simulink model "EvReferenceApplication"  (R2022b)
settings: Solver=FixedStepAuto  StartTime=0  StopTime=inf  FixedStep=TsEV  RelTol=1e-3  EnableMultiTasking=on
StartFcn:
  | load_system('joystick');
  | set_param('joystick', 'SimulationCommand', 'start');
StopFcn:
  | set_param('joystick', 'SimulationCommand', 'stop');
  | % close_system('joystick')
undefined symbols (not defined in the file or in its folder): DiscIntNeverNeededParam, SRE, TsELEC
libraries: simulink x3, autolibshared x2, autolibutils x1, slrealtimeiplib x1, slrealtimeutilitieslib x1
(part 3 of 3)

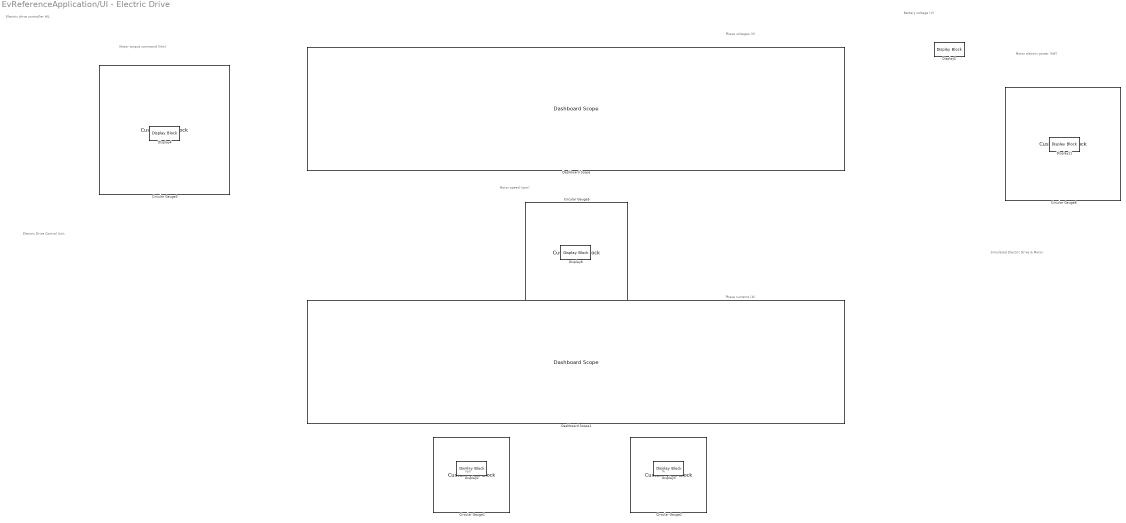
== system EvReferenceApplication/UI - Electric Drive ==
  note: Electric drive controller HIL
  note: kph
  note: %
  note: Motor torque command (Nm)
  note: Phase voltages (V)
  note: Motor speed (rpm)
  note: Battery
      | voltage (V)
  note: Electric Drive
      | Control Unit
  note: Simulated Electric Drive & Motor
  note: Motor electric
      | power (kW)
  note: Phase currents (A)
  Circular Gauge1 : CustomWebBlock  LabelPosition=Hide  ShowInitialText=on  Configuration="{\"components\":[{\"name\":\"CircularScaleComponent\",\"settings\":{\"bounds\":{\"max\":100,\"min\":0,\"tickInterval\":\"auto\"},\"direction\":\"cw\",\"flipLimits\":0,\"innerRadius\":0.75,\"internalTickHeightScaleFactor\":1,\"labelColor\":[228,230,229],\"labelFont\":{\"font\":\"Arial\",\"fontSize\":12},\"labelRadius\":0.528,\"labelTransparency\":1,\"minorTickHeightScaleFactor\":0.2,\"needleImage\":{\"size\":[0,0],\"src\":\"\"},\"needleOffset\":[0,0],\"needleOrientation\":-45,\"needleRotation\":0,\"needleSize\":{\"height\":0,\"width\":0},\"outerRadius\":0.9,\"position\":[0.06486742424242424,0.05627705627705628,0.8917748917748918,0.8787878787878788],\"referencePoint\":\"auto\",\"scaleAngle\":270,\"scaleAngleOffset\":135,\"scaleColors\":[],\"scaleColorsSize\":0.2,\"scaleDirection\":\"CW\",\"scalePosition\":[0,0,1,1],\"showLabels\":1,\"showMinorTicks\":1,\"showSpanLine\":true,\"showTicks\":false,\"tickColor\":[38,38,38],\"tickTransparency\":1,\"valueBarColor\":[0,114,189],\"valueBarPosition\":[0,0,1,1],\"valueBarSize\":0.2,\"valueBarTransparency\":1}},{\"name\":\"BackgroundImageComponent\",\"settings\":{\"image\":{\"size\":[0,0],\"src\":\"default\"},\"position\":[0,0,1,1],\"scaleMode\":\"0\"}},{\"name\":\"ForegroundImageComponent\",\"settings\":{\"image\":{\"size\":[0,0],\"src\":\"default\",\"srcOrientation\":[]},\"isForeground\":1,\"position\":[0,0,1,1],\"scaleMode\":\"0\"}}],\"settings\":{\"BindingType\":\"signal\",\"aspectRatio\":1.032258064516129,\"backgroundColor\":[0,0,0,\"1\"],\"backgroundOffset\":0.14,\"backgroundOpacity\":1,\"direction\":\"cw\",\"fixedAspectRatio\":\"on\",\"flipLimits\":0,\"orientation\":\"horizontal\",\"showBackgroundColor\":false,\"value\":0,\"version\":\"R2022b\"},\"type\":\"CircularGauge\"}"
  Circular Gauge2 : CustomWebBlock  LabelPosition=Hide  ShowInitialText=on  Configuration="{\"components\":[{\"name\":\"CircularScaleComponent\",\"settings\":{\"bounds\":{\"max\":100,\"min\":0,\"tickInterval\":\"auto\"},\"direction\":\"cw\",\"flipLimits\":0,\"innerRadius\":0.75,\"internalTickHeightScaleFactor\":1,\"labelColor\":[228,230,229],\"labelFont\":{\"font\":\"Arial\",\"fontSize\":12},\"labelRadius\":0.528,\"labelTransparency\":1,\"minorTickHeightScaleFactor\":0.2,\"needleImage\":{\"size\":[0,0],\"src\":\"\"},\"needleOffset\":[0,0],\"needleOrientation\":-45,\"needleRotation\":0,\"needleSize\":{\"height\":0,\"width\":0},\"outerRadius\":0.9,\"position\":[0.06486742424242424,0.05627705627705628,0.8917748917748918,0.8787878787878788],\"referencePoint\":\"auto\",\"scaleAngle\":270,\"scaleAngleOffset\":135,\"scaleColors\":[],\"scaleColorsSize\":0.2,\"scaleDirection\":\"CW\",\"scalePosition\":[0,0,1,1],\"showLabels\":1,\"showMinorTicks\":1,\"showSpanLine\":true,\"showTicks\":false,\"tickColor\":[38,38,38],\"tickTransparency\":1,\"valueBarColor\":[0,114,189],\"valueBarPosition\":[0,0,1,1],\"valueBarSize\":0.2,\"valueBarTransparency\":1}},{\"name\":\"BackgroundImageComponent\",\"settings\":{\"image\":{\"size\":[0,0],\"src\":\"default\"},\"position\":[0,0,1,1],\"scaleMode\":\"0\"}},{\"name\":\"ForegroundImageComponent\",\"settings\":{\"image\":{\"size\":[0,0],\"src\":\"default\",\"srcOrientation\":[]},\"isForeground\":1,\"position\":[0,0,1,1],\"scaleMode\":\"0\"}}],\"settings\":{\"BindingType\":\"signal\",\"aspectRatio\":1.032258064516129,\"backgroundColor\":[0,0,0,\"1\"],\"backgroundOffset\":0.14,\"backgroundOpacity\":1,\"direction\":\"cw\",\"fixedAspectRatio\":\"on\",\"flipLimits\":0,\"orientation\":\"horizontal\",\"showBackgroundColor\":false,\"value\":0,\"version\":\"R2022b\"},\"type\":\"CircularGauge\"}"
  Circular Gauge3 : CustomWebBlock  LabelPosition=Hide  ShowInitialText=on  Configuration="{\"components\":[{\"name\":\"CircularScaleComponent\",\"settings\":{\"bounds\":{\"max\":400,\"min\":-300,\"tickInterval\":\"auto\"},\"direction\":\"cw\",\"flipLimits\":0,\"innerRadius\":0.75,\"internalTickHeightScaleFactor\":1,\"labelColor\":[38,38,38],\"labelFont\":{\"font\":\"Arial\",\"fontSize\":12},\"labelRadius\":0.528,\"labelTransparency\":1,\"minorTickHeightScaleFactor\":0.2,\"needleImage\":{\"size\":[0,0],\"src\":\"\"},\"needleOffset\":[0,0],\"needleOrientation\":-45,\"needleRotation\":0,\"needleSize\":{\"height\":0,\"width\":0},\"outerRadius\":0.9,\"position\":[0.06486742424242424,0.05627705627705628,0.8917748917748918,0.8787878787878788],\"referencePoint\":0,\"scaleAngle\":270,\"scaleAngleOffset\":135,\"scaleColors\":[],\"scaleColorsSize\":0.2,\"scaleDirection\":\"CW\",\"scalePosition\":[0,0,1,1],\"showLabels\":1,\"showMinorTicks\":1,\"showSpanLine\":true,\"showTicks\":false,\"tickColor\":[0,114,189],\"tickTransparency\":1,\"valueBarColor\":[0,114,189],\"valueBarPosition\":[0,0,1,1],\"valueBarSize\":0.2,\"valueBarTransparency\":1}},{\"name\":\"BackgroundImageComponent\",\"settings\":{\"image\":{\"size\":[0,0],\"src\":\"default\"},\"position\":[0,0,1,1],\"scaleMode\":\"0\"}},{\"name\":\"ForegroundImageComponent\",\"settings\":{\"image\":{\"size\":[0,0],\"src\":\"default\",\"srcOrientation\":[]},\"isForeground\":1,\"position\":[0,0,1,1],\"scaleMode\":\"0\"}}],\"settings\":{\"BindingType\":\"signal\",\"aspectRatio\":1.032258064516129,\"backgroundColor\":[0,0,0,\"1\"],\"backgroundOffset\":0.14,\"backgroundOpacity\":1,\"direction\":\"cw\",\"fixedAspectRatio\":\"on\",\"flipLimits\":0,\"orientation\":\"horizontal\",\"showBackgroundColor\":false,\"value\":0,\"version\":\"R2022b\"},\"type\":\"CircularGauge\"}"  CustomBackgroundColor="{\"color\":[0.1568627450980392,0.1607843137254902,0.20784313725490197],\"show\":true}"
  Circular Gauge5 : CustomWebBlock  LabelPosition=Hide  ShowInitialText=on  Configuration="{\"components\":[{\"name\":\"CircularScaleComponent\",\"settings\":{\"bounds\":{\"max\":3000,\"min\":0,\"tickInterval\":\"auto\"},\"direction\":\"cw\",\"flipLimits\":0,\"innerRadius\":0.75,\"internalTickHeightScaleFactor\":1,\"labelColor\":[38,38,38],\"labelFont\":{\"font\":\"Arial\",\"fontSize\":12},\"labelRadius\":0.528,\"labelTransparency\":1,\"minorTickHeightScaleFactor\":0.2,\"needleImage\":{\"size\":[0,0],\"src\":\"\"},\"needleOffset\":[0,0],\"needleOrientation\":-45,\"needleRotation\":0,\"needleSize\":{\"height\":0,\"width\":0},\"outerRadius\":0.9,\"position\":[0.06486430921052631,0.05625,0.891633064516129,0.8785978618421053],\"referencePoint\":\"auto\",\"scaleAngle\":270,\"scaleAngleOffset\":135,\"scaleColors\":[],\"scaleColorsSize\":0.2,\"scaleDirection\":\"CW\",\"scalePosition\":[0,0,1,1],\"showLabels\":1,\"showMinorTicks\":1,\"showSpanLine\":true,\"showTicks\":false,\"tickColor\":[0,114,189],\"tickTransparency\":1,\"valueBarColor\":[0,114,189],\"valueBarPosition\":[0,0,1,1],\"valueBarSize\":0.2,\"valueBarTransparency\":1}},{\"name\":\"BackgroundImageComponent\",\"settings\":{\"image\":{\"size\":[0,0],\"src\":\"default\"},\"position\":[0,0,1,1],\"scaleMode\":\"0\"}},{\"name\":\"ForegroundImageComponent\",\"settings\":{\"image\":{\"size\":[0,0],\"src\":\"default\",\"srcOrientation\":[]},\"isForeground\":1,\"position\":[0,0,1,1],\"scaleMode\":\"0\"}}],\"settings\":{\"BindingType\":\"signal\",\"aspectRatio\":1.032258064516129,\"backgroundColor\":[0,0,0,\"1\"],\"backgroundOffset\":0.14,\"backgroundOpacity\":1,\"direction\":\"cw\",\"fixedAspectRatio\":\"on\",\"flipLimits\":0,\"orientation\":\"horizontal\",\"showBackgroundColor\":false,\"value\":0,\"version\":\"R2022b\"},\"type\":\"CircularGauge\"}"  CustomBackgroundColor="{\"color\":[0.1568627450980392,0.1607843137254902,0.20784313725490197],\"show\":true}"
  Circular Gauge8 : CustomWebBlock  LabelPosition=Hide  ShowInitialText=on  Configuration="{\"components\":[{\"name\":\"CircularScaleComponent\",\"settings\":{\"bounds\":{\"max\":200,\"min\":-100,\"tickInterval\":\"auto\"},\"direction\":\"cw\",\"flipLimits\":0,\"innerRadius\":0.75,\"internalTickHeightScaleFactor\":1,\"labelColor\":[38,38,38],\"labelFont\":{\"font\":\"Arial\",\"fontSize\":12},\"labelRadius\":0.528,\"labelTransparency\":1,\"minorTickHeightScaleFactor\":0.2,\"needleImage\":{\"size\":[0,0],\"src\":\"\"},\"needleOffset\":[0,0],\"needleOrientation\":-45,\"needleRotation\":0,\"needleSize\":{\"height\":0,\"width\":0},\"outerRadius\":0.9,\"position\":[0.06487573099415204,0.0561242816091954,0.8917923850574713,0.8786549707602339],\"referencePoint\":0,\"scaleAngle\":270,\"scaleAngleOffset\":135,\"scaleColors\":[],\"scaleColorsSize\":0.2,\"scaleDirection\":\"CW\",\"scalePosition\":[0,0,1,1],\"showLabels\":1,\"showMinorTicks\":1,\"showSpanLine\":true,\"showTicks\":false,\"tickColor\":[0,114,189],\"tickTransparency\":1,\"valueBarColor\":[0,114,189],\"valueBarPosition\":[0,0,1,1],\"valueBarSize\":0.2,\"valueBarTransparency\":1}},{\"name\":\"BackgroundImageComponent\",\"settings\":{\"image\":{\"size\":[0,0],\"src\":\"default\"},\"position\":[0,0,1,1],\"scaleMode\":\"0\"}},{\"name\":\"ForegroundImageComponent\",\"settings\":{\"image\":{\"size\":[0,0],\"src\":\"default\",\"srcOrientation\":[]},\"isForeground\":1,\"position\":[0,0,1,1],\"scaleMode\":\"0\"}}],\"settings\":{\"BindingType\":\"signal\",\"aspectRatio\":1.032258064516129,\"backgroundColor\":[0,0,0,\"1\"],\"backgroundOffset\":0.14,\"backgroundOpacity\":1,\"direction\":\"cw\",\"fixedAspectRatio\":\"on\",\"flipLimits\":0,\"orientation\":\"horizontal\",\"showBackgroundColor\":false,\"value\":0,\"version\":\"R2022b\"},\"type\":\"CircularGauge\"}"  CustomBackgroundColor="{\"color\":[0.1568627450980392,0.1607843137254902,0.20784313725490197],\"show\":true}"
  Dashboard Scope : DashboardScope  TimeSpan=0.050000000000000003  Ymin=-200  Ymax=200  ScaleAtStop=off  UpdateMode=Scroll
  Dashboard Scope1 : DashboardScope  TimeSpan=0.050000000000000003  Ymin=-700  Ymax=700  ScaleAtStop=off  UpdateMode=Scroll
  Display{2..5,8,11} (6 alike) : DisplayBlock  LabelPosition=Hide  Format=Integer  Transparency=1  Opacity=0

== system EvReferenceApplication/Virtual Vehicle ==
  Controllers : Subsystem
      mask Display: image('SystemControllers.png','center')
  Environment : Subsystem
      mask Display: disp(getString(message('autoblks:autoblkVehMask:environ')))
  Longitudinal Driver : Subsystem  Variant=on  VariantControlMode=label  VariantControl=Variant1  LabelModeActiveChoice=0
      mask Display:
      | if strcmp('1',get_param(gcb,'ActiveVariant'))
      |     disp('Open Loop')
      | else
      |     image('LongitudinalDriver.png','center');
      | end
  Passenger Car : Subsystem
      mask Display: image('PassengerVehicle.png','center')
  User Input : Subsystem
      mask Display: image('SpaceMouse.png'); % Use "Edit Image" on toolstrip to change.
  Visualization : Subsystem
      mask Display: disp(getString(message('autoblks:autoblkVehMask:visual')))
  wires:
  Controllers/1(Ctrl) -> Passenger Car/2(Ctrl)
  Passenger Car/1(VehPlnt) -> Longitudinal Driver/2("Vfdbk "), Controllers/2(VehPlnt), Visualization/1(Veh Bus)
  Environment/1(Environment) -> Passenger Car/1(Env)
  Longitudinal Driver/1(" OpCmds") -> Controllers/1(OpCmds)
  User Input/1(speed_cmd) -> Longitudinal Driver/1("Vref ")

== system EvReferenceApplication/Virtual Vehicle/Controllers ==
  OpCmds : Inport
  VehPlnt : Inport  Port=2
  Powertrain Control Input : Subsystem
  Powertrain Control Module (PCM) : Subsystem
  Powertrain Control Output : Subsystem
  Ctrl : Outport  VectorParamsAs1DForOutWhenUnconnected=off
  wires:
  [PtCtrl] -> Ctrl/1
  [OpCmds] -> Powertrain Control Input/1(OpCmds)
  Powertrain Control Output/1(PtCtrl) -> [PtCtrl]
  [VehPlnt] -> Powertrain Control Input/2(VehPlnt)
  VehPlnt/1 -> [VehPlnt]
  OpCmds/1 -> [OpCmds]
  Powertrain Control Input/1(AccelPdl) -> Powertrain Control Module (PCM)/1(AccCmd)
  Powertrain Control Input/2(DecelPdl) -> Powertrain Control Module (PCM)/2(DecCmd)
  Powertrain Control Input/3(VehSpdFdbk) -> Powertrain Control Module (PCM)/3(VehSpdFdbk)
  Powertrain Control Input/4(MotSpd) -> Powertrain Control Module (PCM)/4(MotSpd)
  Powertrain Control Module (PCM)/1(MotTrqCmd) -> Powertrain Control Output/1(MotTrqCmd)
  Powertrain Control Module (PCM)/2(BrakeCmd) -> Powertrain Control Output/2(BrkCmd)
  Powertrain Control Input/5(BMS_Sensors) -> Powertrain Control Module (PCM)/5(BMS_Sensors)
  Powertrain Control Module (PCM)/3(BMS_Info) -> Powertrain Control Output/3(BMS_Info)
  Powertrain Control Module (PCM)/4(BMS_Cmd) -> Powertrain Control Output/4(BMS_Cmd)

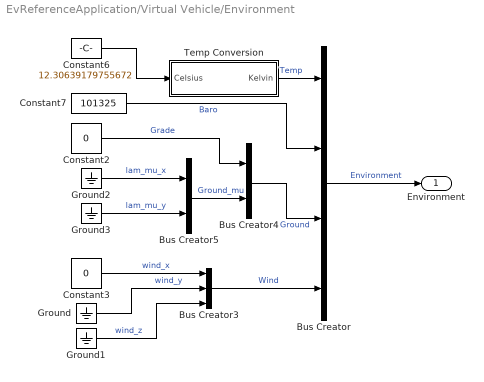
== system EvReferenceApplication/Virtual Vehicle/Environment ==
  Bus Creator : BusCreator  Inputs=4
  Bus Creator3 : BusCreator  Inputs=3
  Bus Creator4 : BusCreator  Inputs=2
  Bus Creator5 : BusCreator  Inputs=2
  Constant2 : Constant  Value=0
  Constant3 : Constant  Value=0
  Constant6 : Constant  Value=12.30639179755672
  Constant7 : Constant  Value=101325
  Ground{,1..3} (4 alike) : Ground
  Temp Conversion : Subsystem
  Environment : Outport  VectorParamsAs1DForOutWhenUnconnected=off
  wires:
  Ground2/1 -> Bus Creator5/1  "lam_mu_x"
  Ground3/1 -> Bus Creator5/2  "lam_mu_y"
  Bus Creator5/1 -> Bus Creator4/2  "Ground_mu"
  Bus Creator4/1 -> Bus Creator/3  "Ground"
  Bus Creator3/1 -> Bus Creator/4  "Wind"
  Constant3/1 -> Bus Creator3/1  "wind_x"
  Ground/1 -> Bus Creator3/2  "wind_y"
  Ground1/1 -> Bus Creator3/3  "wind_z"
  Constant6/1 -> Temp Conversion/1(Celsius)
  Constant2/1 -> Bus Creator4/1  "Grade"
  Bus Creator/1 -> Environment/1  "Environment"
  Constant7/1 -> Bus Creator/2  "Baro"
  Temp Conversion/1(Kelvin) -> Bus Creator/1  "Temp"

== system EvReferenceApplication/Virtual Vehicle/Longitudinal Driver ==
  note: To switch variants, right-click on this subsystem (from one level above) and chose:
      | Variant, Active choice, <your selection>
  "Vref " : Inport
  "Vfdbk " : Inport  Port=2
  Longitudinal Driver : Subsystem  VariantControl=0
      mask Display: image('LongitudinalDriver.png', 'center')
  Open Loop : Subsystem  VariantControl=1
      mask Display: disp('Open Loop')
  " OpCmds" : Outport  VectorParamsAs1DForOutWhenUnconnected=off

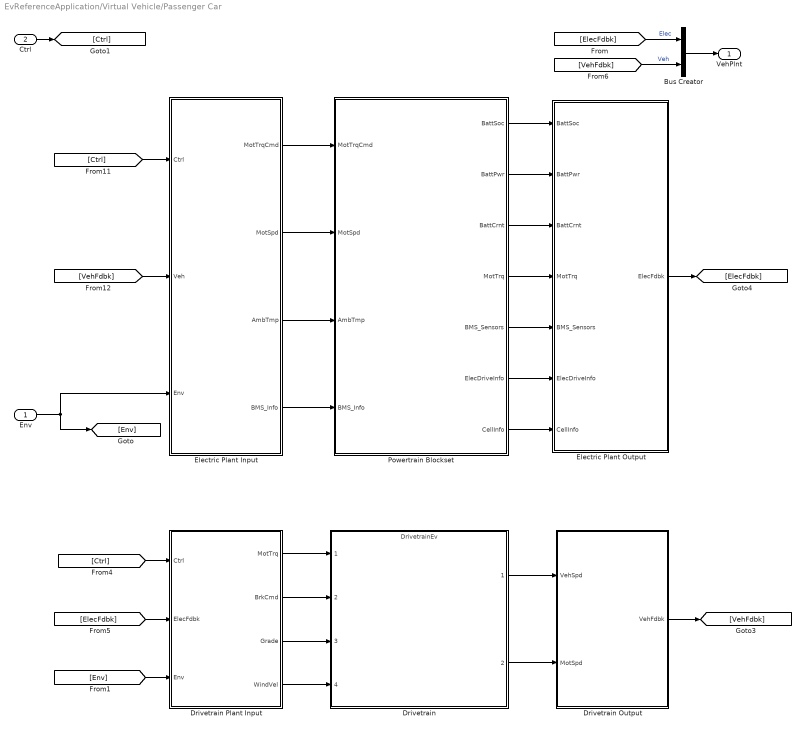
== system EvReferenceApplication/Virtual Vehicle/Passenger Car ==
  Env : Inport
  Ctrl : Inport  Port=2
  Bus Creator : BusCreator  Inputs=2
  Drivetrain : ModelReference  ModelNameDialog=DrivetrainEv.slx  OverrideUsingVariant=Simscape  ModelReferenceVersion=7.0
  Drivetrain Output : Subsystem
  Drivetrain Plant Input : Subsystem
  Electric Plant Input : Subsystem
  Electric Plant Output : Subsystem
  Powertrain Blockset : Subsystem  VariantControl=Powertrain Blockset
  VehPlnt : Outport  VectorParamsAs1DForOutWhenUnconnected=off
  wires:
  Ctrl/1 -> [Ctrl]
  Env/1 -> [Env], Electric Plant Input/3(Env)
  [Ctrl] -> Drivetrain Plant Input/1(Ctrl)
  Bus Creator/1 -> VehPlnt/1
  [VehFdbk] -> Bus Creator/2  "Veh"
  Drivetrain Output/1(VehFdbk) -> [VehFdbk]
  Electric Plant Output/1(ElecFdbk) -> [ElecFdbk]
  [ElecFdbk] -> Bus Creator/1  "Elec"
  [Ctrl] -> Electric Plant Input/1(Ctrl)
  [ElecFdbk] -> Drivetrain Plant Input/2(ElecFdbk)
  [VehFdbk] -> Electric Plant Input/2(Veh)
  Drivetrain Plant Input/2(BrkCmd) -> Drivetrain/2
  Drivetrain Plant Input/1(MotTrq) -> Drivetrain/1
  Drivetrain/2 -> Drivetrain Output/2(MotSpd)
  Drivetrain/1 -> Drivetrain Output/1(VehSpd)
  [Env] -> Drivetrain Plant Input/3(Env)
  Drivetrain Plant Input/3(Grade) -> Drivetrain/3
  Drivetrain Plant Input/4(WindVel) -> Drivetrain/4
  Electric Plant Input/1(MotTrqCmd) -> Powertrain Blockset/1(MotTrqCmd)
  Powertrain Blockset/6(ElecDriveInfo) -> Electric Plant Output/6(ElecDriveInfo)
  Powertrain Blockset/5(BMS_Sensors) -> Electric Plant Output/5(BMS_Sensors)
  Powertrain Blockset/4(MotTrq) -> Electric Plant Output/4(MotTrq)
  Powertrain Blockset/3(BattCrnt) -> Electric Plant Output/3(BattCrnt)
  Powertrain Blockset/2(BattPwr) -> Electric Plant Output/2(BattPwr)
  Powertrain Blockset/1(BattSoc) -> Electric Plant Output/1(BattSoc)
  Electric Plant Input/2(MotSpd) -> Powertrain Blockset/2(MotSpd)
  Electric Plant Input/3(AmbTmp) -> Powertrain Blockset/3(AmbTmp)
  Electric Plant Input/4(BMS_Info) -> Powertrain Blockset/4(BMS_Info)
  Powertrain Blockset/7(CellInfo) -> Electric Plant Output/7(CellInfo)

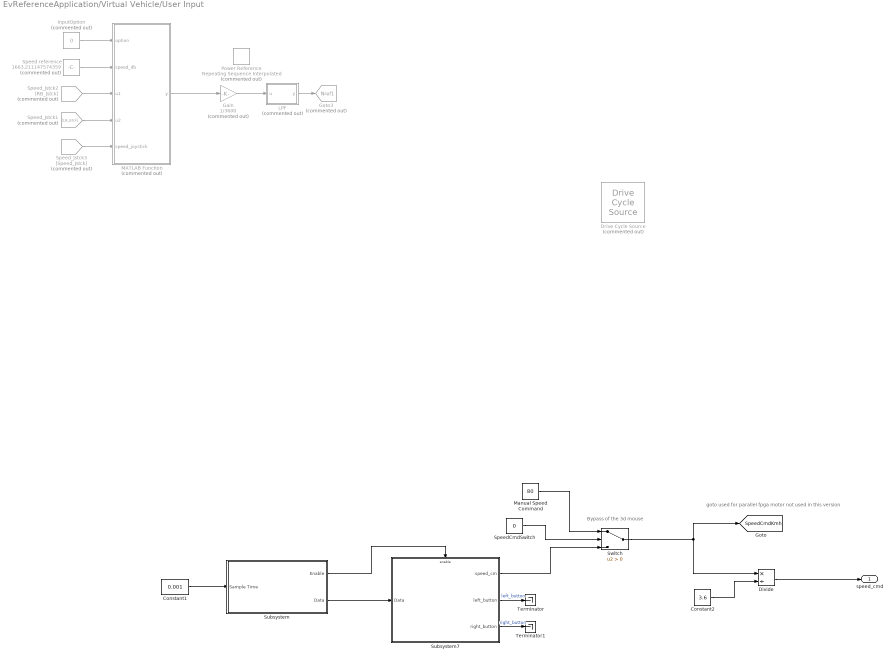
== system EvReferenceApplication/Virtual Vehicle/User Input ==
  note: goto used for parallel fpga motor not used in this version
  note: Bypass of the 3d mouse
  Constant1 : Constant  Value=0.001  SampleTime=0.001
  Constant2 : Constant  Value=3.6  SampleTime=0.001
  Divide : Product  Inputs=*/
  Drive Cycle Source : autolibshared/Drive Cycle Source  Commented=on  cycleVar=FTP75  fileVar=L:\Bauto\matlab\test\toolbox\shared\autoblks\scenario\adac.txt  tfinal="2474  seconds"  cycleRepeat=off  outAccPort=off  outGearPort=off  gearList=No gear data  t_wot1=1  xdot_woto=0  xdot_wot1=26.8*1.1  t_wot2=30  xdot_wot2=0  t_wotend=40  srcUnit=m/s  outUnit=m/s  srcAccUnit=m/s/s  outAccUnit=m/s^2  dt=0  aMode=1  faultOption=off  velBnd=2  velBndUnit=mph  inUnit=m/s  timeBnd=1  failOption=off  stopSim=off  maxFaultCnt=10  maxFaultTime=2  maxTotFaultTime=15  traceOption=off  dtTrace=1  traceWindow=10  lastDCname=FTP75  lastOutUnit=mph  lastDT=0  lastTB=1  lastSB=2  forceCalcBound=off
  Gain : Gain  Commented=on  Gain=1/3600
  Goto3 : Goto  Commented=on  GotoTag=Nref1  TagVisibility=global
  InputOption : Constant  Commented=on  Value=0
  LPF : Subsystem  Commented=on
  MATLAB Function : MATLAB Function  Commented=on  TreatAsAtomicUnit=on
  Manual Speed Command : Constant  Value=80
  Power Reference : simulink/Sources/Repeating Sequence Interpolated  Commented=on  OutValues=[0 0 0.5 0.5 -0.5 -0.5]  TimeValues=[0 5 10 15 25 100]  LookUpMeth=Interpolation-Use End Values  tsamp=TsELEC  OutMin=[]  OutMax=[]  OutDataTypeStr=double  OutputDataTypeScalingMode=double  OutDataType=fixdt(0,8)  OutScaling=2^-10
  Speed reference : Constant  Commented=on  Value=1663.211147574359
  SpeedCmdSwitch : Constant  Value=0
  Speed_Jstck1 : From  Commented=on  GotoTag=LB_Jstck  TagVisibility=global
  Speed_Jstck2 : From  Commented=on  GotoTag=RB_Jstck  TagVisibility=global
  Speed_Jstck3 : From  Commented=on  GotoTag=Speed_Jstck  TagVisibility=global
  Subsystem : Subsystem
  Subsystem7 : Subsystem
  Switch : Switch  Criteria=u2 > Threshold  SaturateOnIntegerOverflow=off  InputSameDT=off
  Terminator : Terminator
  Terminator1 : Terminator
  speed_cmd : Outport
  tag scope: SpeedCmdKmh=global
  wires:
  Gain/1 -> LPF/1(u)
  Speed_Jstck3/1 -> MATLAB Function/5(speed_joystick)
  Subsystem/2(Data) -> Subsystem7/1(Data)
  Constant1/1 -> Subsystem/1(Sample Time)
  Subsystem/1(Enable) -> Subsystem7/Enable
  MATLAB Function/1(y) -> Gain/1
  LPF/1(y) -> Goto3/1
  InputOption/1 -> MATLAB Function/1(option)
  Speed reference/1 -> MATLAB Function/2(speed_db)
  Speed_Jstck2/1 -> MATLAB Function/3(u1)
  Speed_Jstck1/1 -> MATLAB Function/4(u2)
  Subsystem7/2(left_button) -> Terminator/1  "left_button"
  Subsystem7/3(right_button) -> Terminator1/1  "right_button"
  Constant2/1 -> Divide/2
  Divide/1 -> speed_cmd/1
  Manual Speed Command/1 -> Switch/1
  Switch/1 -> [SpeedCmdKmh], Divide/1
  Subsystem7/1(speed_cm) -> Switch/3
  SpeedCmdSwitch/1 -> Switch/2

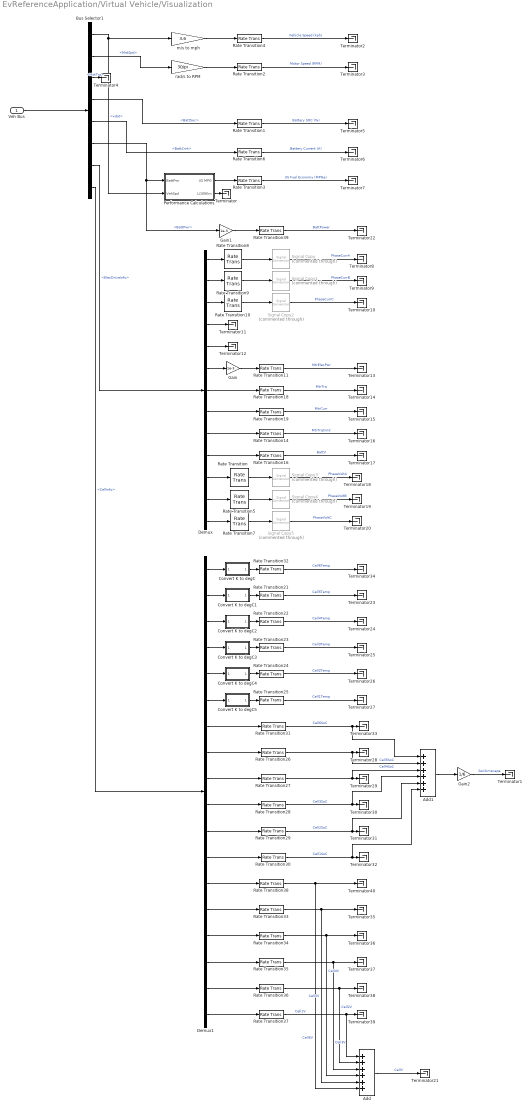
== system EvReferenceApplication/Virtual Vehicle/Visualization ==
  Veh Bus : Inport
  Add : Sum  Inputs=++++++
  Add1 : Sum  Inputs=++++++
  Bus Selector1 : BusSelector  OutputSignals=Veh.xdot,Veh.MotSpd,Elec.MotTrq,Elec.BattSoc,Elec.BattCrnt,Elec.BattPwr,Elec.ElecDriveInfo,Elec.CellInfo
  Convert K to degC : Subsystem
  Convert K to degC1 : Subsystem
  Convert K to degC2 : Subsystem
  Convert K to degC3 : Subsystem
  Convert K to degC4 : Subsystem
  Convert K to degC5 : Subsystem
  Demux : Demux  Outputs=13
  Demux1 : Demux  Outputs=18
  Gain : Gain  Gain=1e-3
  Gain1 : Gain  Gain=1e-3
  Gain2 : Gain  Gain=1/6
  Performance Calculations : Subsystem
  Rate Transition{,5,7..10} (6 alike) : RateTransition  OutPortSampleTime=TsIntrument1kHz
  Rate Transition{1..4,6,11,14,16,18..19} (10 alike) : RateTransition  Deterministic=off  OutPortSampleTime=TsIntrument100Hz
  Rate Transition{21..39} (19 alike) : RateTransition  Deterministic=off  OutPortSampleTime=TsIntrument10Hz
  Signal Copy{,1..5} (6 alike) : SignalConversion  Commented=through  OverrideOpt=on
  Terminator{,1..40} (41 alike) : Terminator
  m/s to mph : Gain  Gain=3.6
  rad/s to RPM : Gain  Gain=30/pi
  wires:
  Bus Selector1/1 -> m/s to mph/1, Performance Calculations/2(VehSpd)  "<xdot>"
  Performance Calculations/1(US MPG) -> Rate Transition3/1
  Performance Calculations/2(L/100Km) -> Terminator/1
  m/s to mph/1 -> Rate Transition4/1
  Bus Selector1/4 -> Rate Transition1/1  "<BattSoc>"
  Rate Transition1/1 -> Terminator5/1  "Battery SOC (%)"
  Rate Transition2/1 -> Terminator3/1  "Motor Speed (RPM)"
  Rate Transition4/1 -> Terminator2/1  "Vehicle Speed (kph)"
  Bus Selector1/2 -> rad/s to RPM/1  "<MotSpd>"
  Bus Selector1/6 -> Gain1/1, Performance Calculations/1(BattPwr)  "<BattPwr>"
  rad/s to RPM/1 -> Rate Transition2/1
  Rate Transition6/1 -> Terminator6/1  "Battery Current (A)"
  Bus Selector1/5 -> Rate Transition6/1  "<BattCrnt>"
  Rate Transition3/1 -> Terminator7/1  "US Fuel Economy (MPGe)"
  Bus Selector1/7 -> Demux/1  "<ElecDriveInfo>"
  Demux/6 -> Gain/1
  Demux/8 -> Rate Transition19/1
  Demux/9 -> Rate Transition14/1
  Demux/1 -> Rate Transition8/1
  Demux/2 -> Rate Transition9/1
  Demux/3 -> Rate Transition10/1
  Rate Transition11/1 -> Terminator13/1  "MtrElecPwr"
  Rate Transition18/1 -> Terminator14/1  "MtrTrq"
  Rate Transition19/1 -> Terminator15/1  "MtrCurr"
  Rate Transition14/1 -> Terminator16/1  "MtrTrqCmd"
  Rate Transition16/1 -> Terminator17/1  "BattV"
  Demux/10 -> Rate Transition16/1
  Demux/11 -> Rate Transition/1
  Demux/12 -> Rate Transition5/1
  Demux/13 -> Rate Transition7/1
  Demux/7 -> Rate Transition18/1
  Gain/1 -> Rate Transition11/1
  Rate Transition32/1 -> Terminator34/1  "Cell6Temp"
  Demux1/1 -> Convert K to degC/1(Kelvin)
  Demux1/2 -> Convert K to degC1/1(Kelvin)
  Rate Transition21/1 -> Terminator23/1  "Cell5Temp"
  Rate Transition22/1 -> Terminator24/1  "Cell4Temp"
  Demux1/3 -> Convert K to degC2/1(Kelvin)
  Demux1/4 -> Convert K to degC3/1(Kelvin)
  Rate Transition23/1 -> Terminator25/1  "Cell3Temp"
  Rate Transition24/1 -> Terminator26/1  "Cell2Temp"
  Demux1/5 -> Convert K to degC4/1(Kelvin)
  Demux1/6 -> Convert K to degC5/1(Kelvin)
  Rate Transition25/1 -> Terminator27/1  "Cell1Temp"
  Rate Transition30/1 -> Add1/6, Terminator32/1  "Cell1SoC"
  Demux1/12 -> Rate Transition30/1
  Demux1/11 -> Rate Transition29/1
  Rate Transition29/1 -> Add1/5, Terminator31/1  "Cell2SoC"
  Rate Transition28/1 -> Add1/4, Terminator30/1  "Cell3SoC"
  Demux1/10 -> Rate Transition28/1
  Demux1/9 -> Rate Transition27/1
  Rate Transition27/1 -> Add1/3, Terminator29/1  "Cell4SoC"
  Rate Transition26/1 -> Add1/2, Terminator28/1  "Cell5SoC"
  Demux1/8 -> Rate Transition26/1
  Demux1/7 -> Rate Transition31/1
  Rate Transition31/1 -> Add1/1, Terminator33/1  "Cell6SoC"
  Rate Transition38/1 -> Add/6, Terminator40/1  "Cell6V"
  Demux1/13 -> Rate Transition38/1
  Demux1/14 -> Rate Transition33/1
  Rate Transition33/1 -> Add/5, Terminator35/1  "Cell5V"
  Rate Transition34/1 -> Add/4, Terminator36/1  "Cell4V"
  Demux1/15 -> Rate Transition34/1
  Demux1/16 -> Rate Transition35/1
  Rate Transition35/1 -> Add/3, Terminator37/1  "Cell3V"
  Rate Transition36/1 -> Add/2, Terminator38/1  "Cell2V"
  Demux1/17 -> Rate Transition36/1
  Demux1/18 -> Rate Transition37/1
  Rate Transition37/1 -> Add/1, Terminator39/1  "Cell1V"
  Bus Selector1/8 -> Demux1/1  "<CellInfo>"
  Convert K to degC/1(Out1) -> Rate Transition32/1
  Convert K to degC1/1(Out1) -> Rate Transition21/1
  Convert K to degC2/1(Out1) -> Rate Transition22/1
  Convert K to degC3/1(Out1) -> Rate Transition23/1
  Convert K to degC4/1(Out1) -> Rate Transition24/1
  Convert K to degC5/1(Out1) -> Rate Transition25/1
  Add/1 -> Terminator21/1  "CellV"
  Gain1/1 -> Rate Transition39/1
  Rate Transition39/1 -> Terminator22/1  "BattPower"
  Bus Selector1/3 -> Terminator4/1  "<MotTrq>"
  Demux/4 -> Terminator11/1
  Demux/5 -> Terminator12/1
  Veh Bus/1 -> Bus Selector1/1
  Signal Copy/1 -> Terminator8/1  "PhaseCurrA"
  Signal Copy1/1 -> Terminator9/1  "PhaseCurrB"
  Signal Copy2/1 -> Terminator10/1  "PhaseCurrC"
  Signal Copy3/1 -> Terminator18/1  "PhaseVoltA"
  Signal Copy4/1 -> Terminator19/1  "PhaseVoltB"
  Signal Copy5/1 -> Terminator20/1  "PhaseVoltC"
  Add1/1 -> Gain2/1
  Gain2/1 -> Terminator1/1  "SocSimscape"
  Rate Transition/1 -> Signal Copy3/1
  Rate Transition5/1 -> Signal Copy4/1
  Rate Transition7/1 -> Signal Copy5/1
  Rate Transition8/1 -> Signal Copy/1
  Rate Transition9/1 -> Signal Copy1/1
  Rate Transition10/1 -> Signal Copy2/1

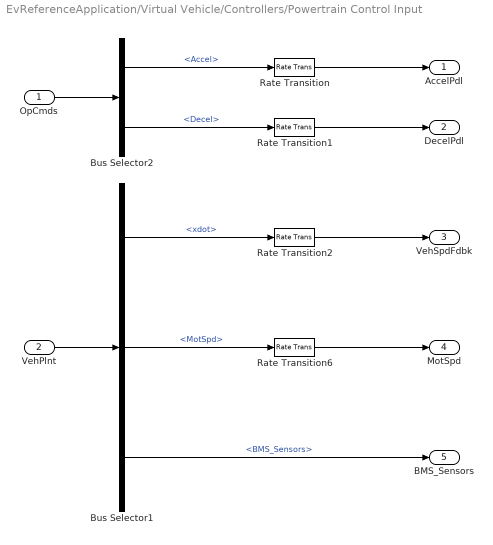
== system EvReferenceApplication/Virtual Vehicle/Controllers/Powertrain Control Input ==
  OpCmds : Inport
  VehPlnt : Inport  Port=2
  Bus Selector1 : BusSelector  OutputSignals=Veh.xdot,Veh.MotSpd,Elec.BMS_Sensors
  Bus Selector2 : BusSelector  OutputSignals=Accel,Decel
  Rate Transition{,1..2,6} (4 alike) : RateTransition  Deterministic=off
  AccelPdl : Outport  VectorParamsAs1DForOutWhenUnconnected=off
  DecelPdl : Outport  Port=2  VectorParamsAs1DForOutWhenUnconnected=off
  VehSpdFdbk : Outport  Port=3  VectorParamsAs1DForOutWhenUnconnected=off
  MotSpd : Outport  Port=4  VectorParamsAs1DForOutWhenUnconnected=off
  BMS_Sensors : Outport  Port=5  OutDataTypeStr=Bus: Sensors  VectorParamsAs1DForOutWhenUnconnected=off
  wires:
  OpCmds/1 -> Bus Selector2/1
  VehPlnt/1 -> Bus Selector1/1
  Bus Selector2/1 -> Rate Transition/1  "<Accel>"
  Bus Selector2/2 -> Rate Transition1/1  "<Decel>"
  Bus Selector1/1 -> Rate Transition2/1  "<xdot>"
  Bus Selector1/2 -> Rate Transition6/1  "<MotSpd>"
  Rate Transition/1 -> AccelPdl/1
  Rate Transition1/1 -> DecelPdl/1
  Rate Transition2/1 -> VehSpdFdbk/1
  Rate Transition6/1 -> MotSpd/1
  Bus Selector1/3 -> BMS_Sensors/1  "<BMS_Sensors>"

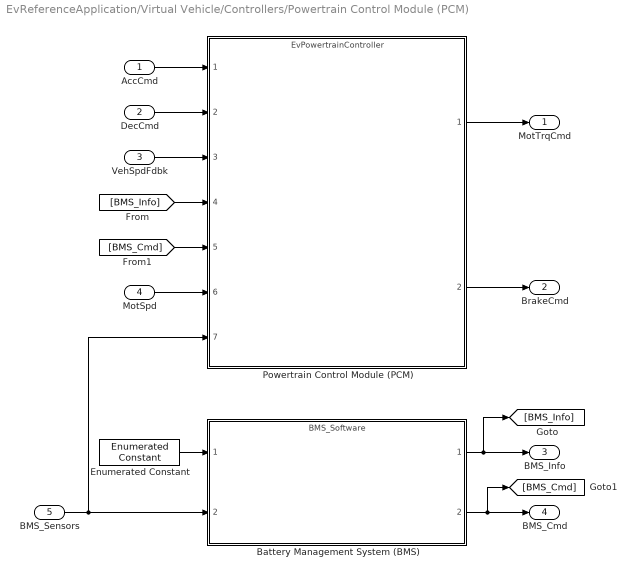
== system EvReferenceApplication/Virtual Vehicle/Controllers/Powertrain Control Module (PCM) ==
  AccCmd : Inport
  DecCmd : Inport  Port=2
  VehSpdFdbk : Inport  Port=3
  MotSpd : Inport  Port=4
  BMS_Sensors : Inport  Port=5  OutDataTypeStr=Bus: Sensors
  Battery Management System (BMS) : ModelReference  ModelNameDialog=BMS_Software.slx  ModelReferenceVersion=4.6
  Enumerated Constant : simulink/Sources/Enumerated Constant  OutDataTypeStr=Enum: SRE  Value=SRE.Driving  SampleTime=inf
  Powertrain Control Module (PCM) : ModelReference  ModelNameDialog=EvPowertrainController.slx  ModelReferenceVersion=5.1
  MotTrqCmd : Outport
  BrakeCmd : Outport  Port=2
  BMS_Info : Outport  Port=3  OutDataTypeStr=Bus: BMS_Info
  BMS_Cmd : Outport  Port=4  OutDataTypeStr=Bus: BMS_Cmd
  wires:
  DecCmd/1 -> Powertrain Control Module (PCM)/2
  Powertrain Control Module (PCM)/1 -> MotTrqCmd/1
  [BMS_Info] -> Powertrain Control Module (PCM)/4
  MotSpd/1 -> Powertrain Control Module (PCM)/6
  VehSpdFdbk/1 -> Powertrain Control Module (PCM)/3
  AccCmd/1 -> Powertrain Control Module (PCM)/1
  Powertrain Control Module (PCM)/2 -> BrakeCmd/1
  Enumerated Constant/1 -> Battery Management System (BMS)/1
  Battery Management System (BMS)/1 -> [BMS_Info], BMS_Info/1
  Battery Management System (BMS)/2 -> [BMS_Cmd], BMS_Cmd/1
  BMS_Sensors/1 -> Powertrain Control Module (PCM)/7, Battery Management System (BMS)/2
  [BMS_Cmd] -> Powertrain Control Module (PCM)/5

== system EvReferenceApplication/Virtual Vehicle/Controllers/Powertrain Control Output ==
  MotTrqCmd : Inport
  BrkCmd : Inport  Port=2
  BMS_Info : Inport  Port=3  OutDataTypeStr=Bus: BMS_Info
  BMS_Cmd : Inport  Port=4  OutDataTypeStr=Bus: BMS_Cmd
  Bus Creator : BusCreator  Inputs=4
  PtCtrl : Outport  VectorParamsAs1DForOutWhenUnconnected=off
  wires:
  BrkCmd/1 -> Bus Creator/2  "BrkCmd"
  Bus Creator/1 -> PtCtrl/1  "PtCtrl"
  MotTrqCmd/1 -> Bus Creator/1  "MotTrqCmd"
  BMS_Info/1 -> Bus Creator/3  "BMS_Info"
  BMS_Cmd/1 -> Bus Creator/4  "BMS_Cmd"

== system EvReferenceApplication/Virtual Vehicle/Environment/Temp Conversion ==
  Celsius : Inport
  Convert degC to K : Subsystem
  Kelvin : Outport
  wires:
  Convert degC to K/1(Out1) -> Kelvin/1
  Celsius/1 -> Convert degC to K/1(Celsius)

== system EvReferenceApplication/Virtual Vehicle/Longitudinal Driver/Longitudinal Driver ==
  Vref : Inport
  Vfdbk : Inport  Port=2
  Bus Selector : BusSelector  OutputSignals=Veh.xdot
  Ground : Ground
  Longitudinal Driver Model : autolibshared/Longitudinal Driver  extAccelOvr=off  extDecelOvr=off  extAccelHld=off  extDecelHld=off  extAccelZero=off  extDecelZero=off  cntrlType=Predictive  shftType=Reverse, Neutral, Drive  velUnits=m/s  gearOut=off  Kp=1  Ki=1  Kff=0  Kg=0  VehVelVec=[0 100]  KffVec=[.1 .1]  KpVec=[10 10]  KiVec=[5 5]  KgVec=[0 0]  m=1645  Kpt=450*9.04/0.324  tau=0.12  L=4  aR=30.3/3875  bR=0.21290*4.44822/0.44704  cR=0.01278*4.44822/0.44704^2  g=9.81  vnom=1  Kaw=0  tauerr=0  tauPt=2  GearInit=0  tShift=.1  pdlVec=[0.1 0.4 0.5 0.9]  upShftTbl=[-1 12.9375 26.4375 39.9375 51.18749999999999 62.4375 72.84375 83.25;-1 16.3125 29.8125 43.3125 54.5624 65.8125 76.78125 87.75;-1 19.6875 33.1875 46.68749999999999 57.9375 69.1875 80.71875 92.25;-1 33 52.5 77.25 100.5 138.75 161.875 185]  dwnShftTbl=[1 9.5625 23.0625 36.5625 47.8125 59.0625 68.90625 78.75;1 12.9375 26.4375 39.9375 51.18749999999999 62.4375 72.84375 83.25;1 16.3125 29.8125 43.3125 54.562499 65.8125 76.78125 87.75;1 19.6875 33.1875 46.68749999999999 57.9375 69.1875 80.71875 92.25]  tClutch=.5  tRev=.5  tPark=120  aMode=1  UpGearVec="[0  1  2  3  4  5  6  7]"  DownGearVec="[1  2  3  4  5  6  7  8]"
  Terminator : Terminator
  Terminator1 : Terminator
  OpCmds : Outport  VectorParamsAs1DForOutWhenUnconnected=off
  wires:
  Bus Selector/1 -> Longitudinal Driver Model/2  "<xdot>"
  Vref/1 -> Longitudinal Driver Model/1  "xdotref"
  Vfdbk/1 -> Bus Selector/1
  Longitudinal Driver Model/2 -> Terminator/1  "Acc"
  Longitudinal Driver Model/3 -> Terminator1/1  "Dec"
  Ground/1 -> Longitudinal Driver Model/3
  Longitudinal Driver Model/1 -> OpCmds/1  "Info"

== system EvReferenceApplication/Virtual Vehicle/Longitudinal Driver/Open Loop ==
  note: This subsystem is provided to disable the driver subsystem and expose the driver interface.
      |
      | The interface can:
      | - be connected with dashboard UI blocks or 3rd party hardware
      | - provide application specific pre-programmed event or time based signals
      | - be driven by recorded operator signals for tuning, troubleshooting and model validation
  Bus Creator2 : BusCreator  Inputs=8
  Constant{1..4} (4 alike) : Constant  Value=0
  Ground{,1..3} (4 alike) : Ground
  OpCmds : Outport  VectorParamsAs1DForOutWhenUnconnected=off
  wires:
  Ground3/1 -> Bus Creator2/8  "ErrMin"
  Ground1/1 -> Bus Creator2/6  "ErrSqrSum"
  Bus Creator2/1 -> OpCmds/1  "Info"
  Ground2/1 -> Bus Creator2/7  "ErrMax"
  Constant1/1 -> Bus Creator2/1  "Accel"
  Constant3/1 -> Bus Creator2/3  "Gear"
  Constant2/1 -> Bus Creator2/2  "Decel"
  Ground/1 -> Bus Creator2/5  "Err"
  Constant4/1 -> Bus Creator2/4  "Clutch"

== system EvReferenceApplication/Virtual Vehicle/Passenger Car/Drivetrain Output ==
  VehSpd : Inport
  MotSpd : Inport  Port=2
  Bus Creator1 : BusCreator  Inputs=2
  VehFdbk : Outport  VectorParamsAs1DForOutWhenUnconnected=off
  wires:
  Bus Creator1/1 -> VehFdbk/1  "VehFdbk"
  VehSpd/1 -> Bus Creator1/1
  MotSpd/1 -> Bus Creator1/2  "MotSpd"

== system EvReferenceApplication/Virtual Vehicle/Passenger Car/Drivetrain Plant Input ==
  Ctrl : Inport
  ElecFdbk : Inport  Port=2
  Env : Inport  Port=3
  Bus Selector : BusSelector  OutputSignals=BrkCmd
  Bus Selector1 : BusSelector  OutputSignals=MotTrq
  Bus Selector3 : BusSelector  OutputSignals=Ground.Grade,Wind.wind_x
  First Order Hold : FirstOrderHold  ErrorTolerance=inf
  Rate Transition6 : RateTransition  Deterministic=off
  Rate Transition7 : RateTransition  Deterministic=off
  MotTrq : Outport  VectorParamsAs1DForOutWhenUnconnected=off
  BrkCmd : Outport  Port=2  VectorParamsAs1DForOutWhenUnconnected=off
  Grade : Outport  Port=3  VectorParamsAs1DForOutWhenUnconnected=off
  WindVel : Outport  Port=4  VectorParamsAs1DForOutWhenUnconnected=off
  wires:
  Ctrl/1 -> Bus Selector/1
  Bus Selector/1 -> First Order Hold/1  "<BrkCmd>"
  First Order Hold/1 -> BrkCmd/1  "BrkCmd"
  ElecFdbk/1 -> Bus Selector1/1
  Bus Selector1/1 -> MotTrq/1  "<MotTrq>"
  Env/1 -> Bus Selector3/1
  Rate Transition6/1 -> Grade/1  "Grade"
  Rate Transition7/1 -> WindVel/1  "WindVel"
  Bus Selector3/1 -> Rate Transition6/1  "<Grade>"
  Bus Selector3/2 -> Rate Transition7/1  "<wind_x>"

== system EvReferenceApplication/Virtual Vehicle/Passenger Car/Electric Plant Input ==
  Ctrl : Inport
  Veh : Inport  Port=2
  Env : Inport  Port=3
  Bus Selector : BusSelector  OutputSignals=MotTrqCmd,BMS_Info
  Bus Selector1 : BusSelector  OutputSignals=MotSpd
  Bus Selector2 : BusSelector  OutputSignals=Temp
  First Order Hold : FirstOrderHold  ErrorTolerance=inf
  MotTrqCmd : Outport  VectorParamsAs1DForOutWhenUnconnected=off
  MotSpd : Outport  Port=2  VectorParamsAs1DForOutWhenUnconnected=off
  AmbTmp : Outport  Port=3  VectorParamsAs1DForOutWhenUnconnected=off
  BMS_Info : Outport  Port=4  OutDataTypeStr=Bus: BMS_Info  VectorParamsAs1DForOutWhenUnconnected=off
  wires:
  First Order Hold/1 -> MotTrqCmd/1  "MotTrqCmd"
  Ctrl/1 -> Bus Selector/1
  Bus Selector/1 -> First Order Hold/1  "<MotTrqCmd>"
  Veh/1 -> Bus Selector1/1
  Bus Selector1/1 -> MotSpd/1  "<MotSpd>"
  Env/1 -> Bus Selector2/1
  Bus Selector2/1 -> AmbTmp/1  "<Temp>"
  Bus Selector/2 -> BMS_Info/1  "<BMS_Info>"

== system EvReferenceApplication/Virtual Vehicle/Passenger Car/Electric Plant Output ==
  BattSoc : Inport
  BattPwr : Inport  Port=2
  BattCrnt : Inport  Port=3
  MotTrq : Inport  Port=4
  BMS_Sensors : Inport  Port=5  OutDataTypeStr=Bus: Sensors
  ElecDriveInfo : Inport  Port=6
  CellInfo : Inport  Port=7
  Bus Creator1 : BusCreator  Inputs=7
  ElecFdbk : Outport  VectorParamsAs1DForOutWhenUnconnected=off
  wires:
  Bus Creator1/1 -> ElecFdbk/1  "ElecFdbk"
  BattPwr/1 -> Bus Creator1/2
  BattCrnt/1 -> Bus Creator1/3
  MotTrq/1 -> Bus Creator1/4
  BMS_Sensors/1 -> Bus Creator1/5
  BattSoc/1 -> Bus Creator1/1
  ElecDriveInfo/1 -> Bus Creator1/6
  CellInfo/1 -> Bus Creator1/7

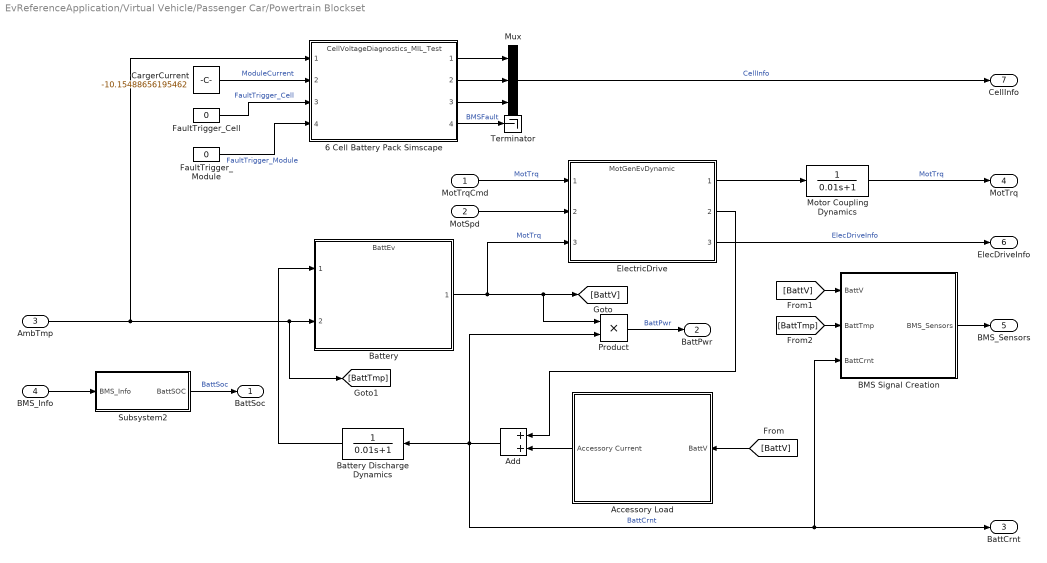
== system EvReferenceApplication/Virtual Vehicle/Passenger Car/Powertrain Blockset ==
  MotTrqCmd : Inport
  MotSpd : Inport  Port=2
  AmbTmp : Inport  Port=3  Unit=K
  BMS_Info : Inport  Port=4  OutDataTypeStr=Bus: BMS_Info
  6 Cell Battery Pack Simscape : ModelReference  ModelNameDialog=CellVoltageDiagnostics_MIL_Test.slx  SimulationMode=Normal  ModelReferenceVersion=7.1
  Accessory Load : Subsystem
  Add : Sum
  BMS Signal Creation : Subsystem
  Battery : ModelReference  ModelNameDialog=BattEv.slx  SimulationMode=Normal  ModelReferenceVersion=8.32
  Battery Discharge Dynamics : TransferFcn  Denominator=[0.01 1]
  CargerCurrent : Constant  Value=-10.15488656195462
  ElectricDrive : ModelReference  ModelNameDialog=MotGenEvDynamic.slx  SimulationMode=Normal  ModelReferenceVersion=8.72
  FaultTrigger_Cell : Constant  Value=0  OutDataTypeStr=boolean
  FaultTrigger_Module : Constant  Value=0  OutDataTypeStr=boolean
  Motor Coupling Dynamics : TransferFcn  Denominator=[0.01 1]
  Mux : Mux  Inputs=3
  Product : Product
  Subsystem2 : Subsystem
  Terminator : Terminator
  BattSoc : Outport
  BattPwr : Outport  Port=2  VectorParamsAs1DForOutWhenUnconnected=off
  BattCrnt : Outport  Port=3  VectorParamsAs1DForOutWhenUnconnected=off
  MotTrq : Outport  Port=4  VectorParamsAs1DForOutWhenUnconnected=off
  BMS_Sensors : Outport  Port=5  OutDataTypeStr=Bus: Sensors  VectorParamsAs1DForOutWhenUnconnected=off
  ElecDriveInfo : Outport  Port=6  VectorParamsAs1DForOutWhenUnconnected=off
  CellInfo : Outport  Port=7
  wires:
  Product/1 -> BattPwr/1  "BattPwr"
  Battery Discharge Dynamics/1 -> Battery/1
  ElectricDrive/1 -> Motor Coupling Dynamics/1
  Motor Coupling Dynamics/1 -> MotTrq/1  "MotTrq"
  Accessory Load/1(Accessory Current) -> Add/2
  ElectricDrive/2 -> Add/1
  [BattV] -> Accessory Load/1(BattV)
  Add/1 -> Battery Discharge Dynamics/1, BattCrnt/1, BMS Signal Creation/3(BattCrnt), Product/2  "BattCrnt"
  [BattV] -> BMS Signal Creation/1(BattV)
  [BattTmp] -> BMS Signal Creation/2(BattTmp)
  BMS Signal Creation/1(BMS_Sensors) -> BMS_Sensors/1
  AmbTmp/1 -> 6 Cell Battery Pack Simscape/1, [BattTmp], Battery/2
  BMS_Info/1 -> Subsystem2/1(BMS_Info)
  Subsystem2/1(BattSOC) -> BattSoc/1  "BattSoc"
  ElectricDrive/3 -> ElecDriveInfo/1  "ElecDriveInfo"
  6 Cell Battery Pack Simscape/3 -> Mux/3
  6 Cell Battery Pack Simscape/2 -> Mux/2
  6 Cell Battery Pack Simscape/1 -> Mux/1
  CargerCurrent/1 -> 6 Cell Battery Pack Simscape/2  "ModuleCurrent"
  Mux/1 -> CellInfo/1  "CellInfo"
  6 Cell Battery Pack Simscape/4 -> Terminator/1  "BMSFault"
  FaultTrigger_Cell/1 -> 6 Cell Battery Pack Simscape/3  "FaultTrigger_Cell"
  FaultTrigger_Module/1 -> 6 Cell Battery Pack Simscape/4  "FaultTrigger_Module"
  MotSpd/1 -> ElectricDrive/2
  MotTrqCmd/1 -> ElectricDrive/1  "MotTrq"
  Battery/1 -> [BattV], Product/1, ElectricDrive/3  "MotTrq"

== system EvReferenceApplication/Virtual Vehicle/User Input/LPF ==
  u : Inport
  Discrete-Time Integrator : DiscreteIntegrator  gainval=20  SampleTime=TsELEC  ICPrevOutput=DiscIntNeverNeededParam  ICPrevScaledInput=DiscIntNeverNeededParam
  Sum : Sum  Inputs=|+-
  y : Outport
  wires:
  Sum/1 -> Discrete-Time Integrator/1
  Discrete-Time Integrator/1 -> y/1, Sum/2
  u/1 -> Sum/1

== system EvReferenceApplication/Virtual Vehicle/User Input/Subsystem ==
  Sample Time : Inport
  Compare To Constant : simulink/Logic and Bit Operations/Compare To Constant  relop===  const=24  OutDataTypeStr=boolean
  Constant : Constant
  Data Type Conversion : DataTypeConversion  OutDataTypeStr=boolean  SaturateOnIntegerOverflow=off  RndMeth=Floor
  Subtract : Sum  Inputs=+-
  Terminator : Terminator
  UDP Receive : slrealtimeiplib/UDP Receive  useHostTargetConn=on  ipAddress='192.168.7.5'  localPort=25000  rcvWidth=24  rcvFmAny=off  fmAddress='172.16.19.80'  sampleTime=-1  enableMessage=off  maxPackets=1
  Unit Delay : UnitDelay  SampleTime=-1  HasFrameUpgradeWarning=on
  While Iterator : WhileIterator  WhileBlockType=do-while  ShowIterationPort=on
  Enable : Outport
  Data : Outport  Port=2
  wires:
  Compare To Constant/1 -> While Iterator/1
  UDP Receive/1 -> Unit Delay/1
  Constant/1 -> Subtract/2
  UDP Receive/2 -> Compare To Constant/1
  While Iterator/1 -> Subtract/1
  Sample Time/1 -> Terminator/1
  Subtract/1 -> Data Type Conversion/1
  Unit Delay/1 -> Data/1
  Data Type Conversion/1 -> Enable/1

== system EvReferenceApplication/Virtual Vehicle/User Input/Subsystem7 ==
  Data : Inport
  Enable : EnablePort
  Byte Unpacking : slrealtimeutilitieslib/Byte Unpacking  MaskUnpackedDataTypes={'double','double','double'}  MaskUnpackedDataSizes={[1],[1],[1]}  MaskAlignment=1
  speed_cm : Outport
  left_button : Outport  Port=2
  right_button : Outport  Port=3
  wires:
  Data/1 -> Byte Unpacking/1
  Byte Unpacking/1 -> speed_cm/1
  Byte Unpacking/2 -> left_button/1
  Byte Unpacking/3 -> right_button/1

== system EvReferenceApplication/Virtual Vehicle/Visualization/Convert K to degC ==
  Kelvin : Inport
  Constant1 : Constant  Value=273.15
  Sum : Sum  Inputs=+-
  Out1 : Outport
  wires:
  Kelvin/1 -> Sum/1
  Constant1/1 -> Sum/2
  Sum/1 -> Out1/1

== system EvReferenceApplication/Virtual Vehicle/Visualization/Convert K to degC1 ==
  Kelvin : Inport
  Constant1 : Constant  Value=273.15
  Sum : Sum  Inputs=+-
  Out1 : Outport
  wires:
  Sum/1 -> Out1/1
  Constant1/1 -> Sum/2
  Kelvin/1 -> Sum/1

== system EvReferenceApplication/Virtual Vehicle/Visualization/Convert K to degC2 ==
  Kelvin : Inport
  Constant1 : Constant  Value=273.15
  Sum : Sum  Inputs=+-
  Out1 : Outport
  wires:
  Kelvin/1 -> Sum/1
  Constant1/1 -> Sum/2
  Sum/1 -> Out1/1

== system EvReferenceApplication/Virtual Vehicle/Visualization/Convert K to degC3 ==
  Kelvin : Inport
  Constant1 : Constant  Value=273.15
  Sum : Sum  Inputs=+-
  Out1 : Outport
  wires:
  Sum/1 -> Out1/1
  Constant1/1 -> Sum/2
  Kelvin/1 -> Sum/1

== system EvReferenceApplication/Virtual Vehicle/Visualization/Convert K to degC4 ==
  Kelvin : Inport
  Constant1 : Constant  Value=273.15
  Sum : Sum  Inputs=+-
  Out1 : Outport
  wires:
  Kelvin/1 -> Sum/1
  Constant1/1 -> Sum/2
  Sum/1 -> Out1/1

== system EvReferenceApplication/Virtual Vehicle/Visualization/Convert K to degC5 ==
  Kelvin : Inport
  Constant1 : Constant  Value=273.15
  Sum : Sum  Inputs=+-
  Out1 : Outport
  wires:
  Sum/1 -> Out1/1
  Constant1/1 -> Sum/2
  Kelvin/1 -> Sum/1

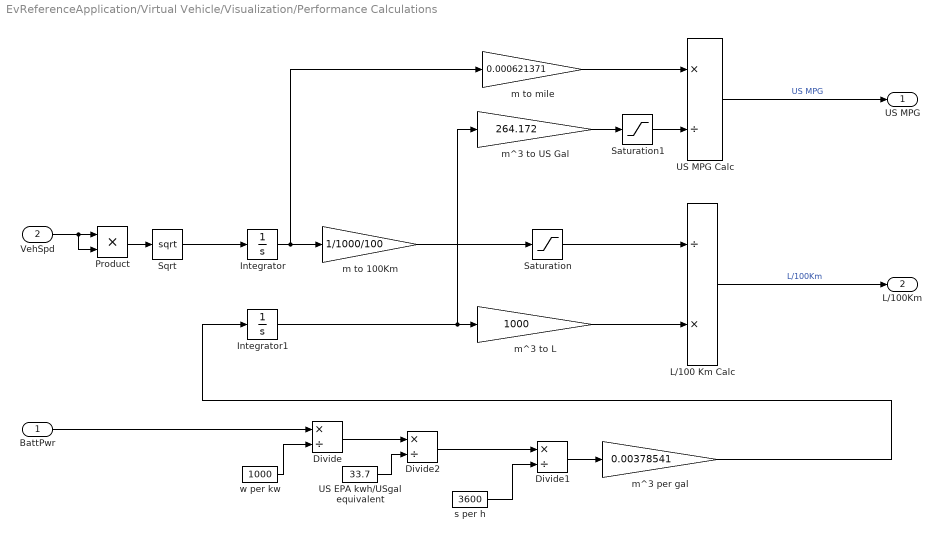
== system EvReferenceApplication/Virtual Vehicle/Visualization/Performance Calculations ==
  BattPwr : Inport
  VehSpd : Inport  Port=2
  Divide : Product  Inputs=*/
  Divide1 : Product  Inputs=*/
  Divide2 : Product  Inputs=*/
  Integrator : Integrator
  Integrator1 : Integrator
  L/100 Km Calc : Product  Inputs=/*
  Product : Product
  Saturation : Saturate  UpperLimit=Inf  LowerLimit=0.001  ZeroCross=off
  Saturation1 : Saturate  UpperLimit=Inf  LowerLimit=1e-3  ZeroCross=off
  Sqrt : Sqrt
  US EPA kwh/USgal equivalent : Constant  Value=33.7
  US MPG Calc : Product  Inputs=*/
  m to 100Km : Gain  Gain=1/1000/100
  m to mile : Gain  Gain=0.000621371
  m^3 per gal : Gain  Gain=0.00378541
  m^3 to L : Gain  Gain=1000
  m^3 to US Gal : Gain  Gain=264.172
  s per h : Constant  Value=3600
  w per kw : Constant  Value=1000
  US MPG : Outport  VectorParamsAs1DForOutWhenUnconnected=off
  L/100Km : Outport  Port=2  VectorParamsAs1DForOutWhenUnconnected=off
  wires:
  m^3 to US Gal/1 -> Saturation1/1
  m^3 to L/1 -> L/100 Km Calc/2
  Integrator/1 -> m to mile/1, m to 100Km/1
  m to mile/1 -> US MPG Calc/1
  Integrator1/1 -> m^3 to US Gal/1, m^3 to L/1
  Saturation/1 -> L/100 Km Calc/1
  m to 100Km/1 -> Saturation/1
  L/100 Km Calc/1 -> L/100Km/1  "L/100Km"
  Saturation1/1 -> US MPG Calc/2
  US MPG Calc/1 -> US MPG/1  "US MPG"
  w per kw/1 -> Divide/2
  Divide/1 -> Divide2/1
  Divide2/1 -> Divide1/1
  s per h/1 -> Divide1/2
  Divide1/1 -> m^3 per gal/1
  m^3 per gal/1 -> Integrator1/1
  US EPA kwh/USgal equivalent/1 -> Divide2/2
  BattPwr/1 -> Divide/1
  Sqrt/1 -> Integrator/1
  Product/1 -> Sqrt/1
  VehSpd/1 -> Product/2, Product/1

== system EvReferenceApplication/Virtual Vehicle/Environment/Temp Conversion/Convert degC to K ==
  Celsius : Inport
  Constant1 : Constant  Value=273.15
  Sum : Sum
  Out1 : Outport
  wires:
  Celsius/1 -> Sum/1
  Constant1/1 -> Sum/2
  Sum/1 -> Out1/1

== system EvReferenceApplication/Virtual Vehicle/Passenger Car/Powertrain Blockset/Accessory Load ==
  BattV : Inport
  Accessory Load W : Constant  Value=0
  Divide : Product  Inputs=*/
  div0protect - poly : autolibutils/div0protect - poly  thresh=.01  ZeroCross=off  ZeroCross1=off  aMode=aMode
  Accessory Current : Outport
  wires:
  BattV/1 -> div0protect - poly/1
  Accessory Load W/1 -> Divide/1
  Divide/1 -> Accessory Current/1
  div0protect - poly/1 -> Divide/2

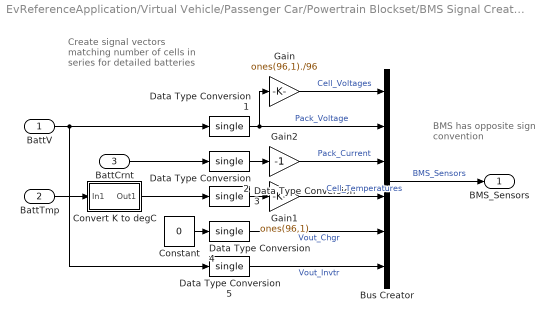
== system EvReferenceApplication/Virtual Vehicle/Passenger Car/Powertrain Blockset/BMS Signal Creation ==
  note: Create signal vectors
      | matching number of
      | cells in series for
      | detailed batteries
  note: BMS has opposite
      | sign convention
  BattV : Inport
  BattTmp : Inport  Port=2
  BattCrnt : Inport  Port=3
  Bus Creator : BusCreator  Inputs=6  OutDataTypeStr=Bus: Sensors  NonVirtualBus=on
      settings: InheritFromInputs=off
  Constant : Constant  Value=0
  Convert K to degC : Subsystem
  Data Type Conversion{1..5} (5 alike) : DataTypeConversion  OutDataTypeStr=single  SaturateOnIntegerOverflow=off  RndMeth=Floor
  Gain : Gain  Gain=ones(96,1)./96
  Gain1 : Gain  Gain=ones(96,1)
  Gain2 : Gain  Gain=-1
  BMS_Sensors : Outport
  wires:
  Gain1/1 -> Bus Creator/4  "Cell_Temperatures"
  Data Type Conversion4/1 -> Bus Creator/5  "Vout_Chgr"
  Gain2/1 -> Bus Creator/3  "Pack_Current"
  Data Type Conversion5/1 -> Bus Creator/6  "Vout_Invtr"
  Data Type Conversion2/1 -> Gain2/1
  Gain/1 -> Bus Creator/1  "Cell_Voltages"
  Data Type Conversion3/1 -> Gain1/1
  Data Type Conversion1/1 -> Gain/1, Bus Creator/2  "Pack_Voltage"
  BattTmp/1 -> Convert K to degC/1(In1)
  BattCrnt/1 -> Data Type Conversion2/1
  Constant/1 -> Data Type Conversion4/1
  BattV/1 -> Data Type Conversion1/1, Data Type Conversion5/1
  Bus Creator/1 -> BMS_Sensors/1  "BMS_Sensors"
  Convert K to degC/1(Out1) -> Data Type Conversion3/1

== system EvReferenceApplication/Virtual Vehicle/Passenger Car/Powertrain Blockset/Subsystem2 ==
  In Bus Element : Inport  PortName=BMS_Info  Element=SOC
  Bus Selector : BusSelector  OutputSignals=SOC_CC
  Data Type Conversion : DataTypeConversion  SaturateOnIntegerOverflow=off  RndMeth=Floor
  Rate Transition : RateTransition  Commented=through
  convert2percent : Gain  Gain=100
  BattSOC : Outport
  wires:
  In Bus Element/1 -> Bus Selector/1
  convert2percent/1 -> Data Type Conversion/1
  Bus Selector/1 -> convert2percent/1  "<SOC_CC>"
  Data Type Conversion/1 -> Rate Transition/1
  Rate Transition/1 -> BattSOC/1

== system EvReferenceApplication/Virtual Vehicle/Passenger Car/Powertrain Blockset/BMS Signal Creation/Convert K to degC ==
  In1 : Inport
  Constant1 : Constant  Value=273.15
  Sum : Sum  Inputs=+-
  Out1 : Outport
  wires:
  In1/1 -> Sum/1
  Constant1/1 -> Sum/2
  Sum/1 -> Out1/1

== matlab function EvReferenceApplication/Virtual Vehicle/User Input/MATLAB Function ==
  data: option input; speed_db input; u1 input; y output; u2 input; speed_joystick input
function y = fcn(option,speed_db,u1,u2,speed_joystick)

if option
    y=speed_db;
else
    if u1
        y = 1600;
    elseif u2
        y = -1600;
    else
        y = speed_joystick;
    end
end
